simulink library "kinematics"  (R2025b)
settings: Solver=VariableStepAuto  StartTime=0.0  StopTime=10.0  RelTol=1e-3
values from neighbouring files (symbols this model uses):
  A_BN0 = eye(3)    [lab_7_task_1.m]    (also in lab_7_task_3.m)
settings Model: Creator=nicol  LastModifiedBy=nicol

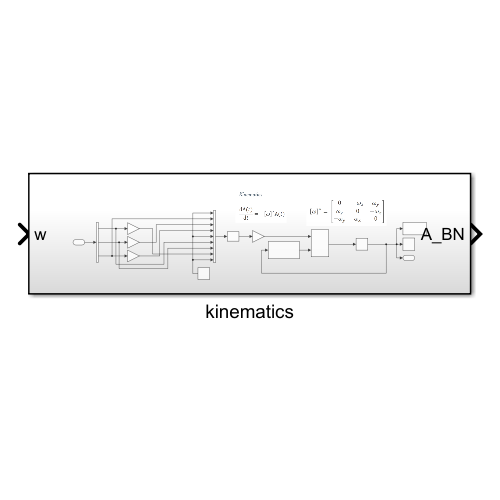
[thumbnail: Simulink's stored preview of the top-level diagram]
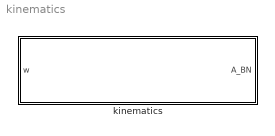
== system kinematics ==
  kinematics : Subsystem

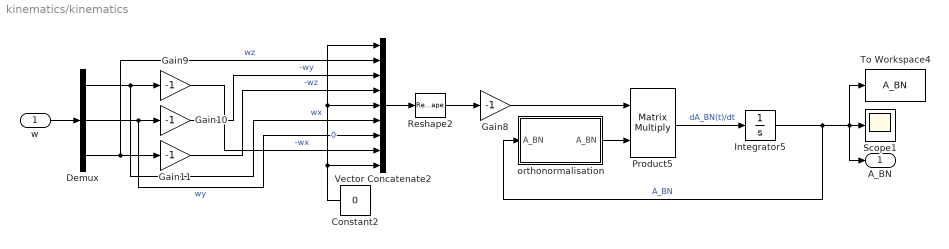
== system kinematics/kinematics ==
  w : Inport
  Constant2 : Constant  Value=0
  Demux : Demux  Outputs=3
  Gain{8..11} (4 alike) : Gain  Gain=-1
  Integrator5 : Integrator  InitialCondition=A_BN0
  Product5 : Product  Multiplication=Matrix(*)
  Reshape2 : Reshape  OutputDimensionality=Customize  OutputDimensions=[3,3]
  Scope1 : Scope
      settings: ActiveDisplayYMinimum=-1.2499999998899596  ActiveDisplayYMaximum=1.2499999999877733
  To Workspace4 : ToWorkspace  VariableName=A_BN  SaveFormat=Timeseries  SampleTime=-1
  Vector Concatenate2 : Concatenate  NumInputs=9
  orthonormalisation : Subsystem
  A_BN : Outport
  wires:
  orthonormalisation/1(" A_BN") -> Product5/2
  w/1 -> Demux/1
  Gain9/1 -> Vector Concatenate2/8  "-wx"
  Constant2/1 -> Vector Concatenate2/9, Vector Concatenate2/5, Vector Concatenate2/1  "0"
  Demux/3 -> Gain11/1, Vector Concatenate2/2  "wz"
  Vector Concatenate2/1 -> Reshape2/1
  Demux/2 -> Gain10/1, Vector Concatenate2/7  "wy"
  Gain10/1 -> Vector Concatenate2/3  "-wy"
  Reshape2/1 -> Gain8/1
  Demux/1 -> Gain9/1, Vector Concatenate2/6  "wx"
  Gain8/1 -> Product5/1
  Integrator5/1 -> orthonormalisation/1(A_BN), Scope1/1, To Workspace4/1, A_BN/1  "A_BN"
  Gain11/1 -> Vector Concatenate2/4  "-wz"
  Product5/1 -> Integrator5/1  "dA_BN(t)/dt"

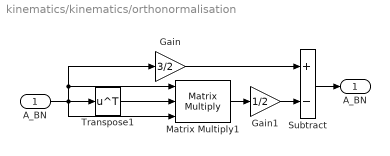
== system kinematics/kinematics/orthonormalisation ==
  A_BN : Inport
  Gain : Gain  Gain=3/2
  Gain1 : Gain  Gain=1/2
  Matrix Multiply1 : Product  Inputs=3  Multiplication=Matrix(*)
  Subtract : Sum  Inputs=+-
  Transpose1 : Math  Operator=transpose
  " A_BN" : Outport
  wires:
  A_BN/1 -> Matrix Multiply1/3, Transpose1/1, Gain/1, Matrix Multiply1/1
  Subtract/1 -> " A_BN"/1
  Gain1/1 -> Subtract/2
  Matrix Multiply1/1 -> Gain1/1
  Transpose1/1 -> Matrix Multiply1/2
  Gain/1 -> Subtract/1
